simulink library "Custom_Valve_Orifices_Lib"  (R2013a)
settings: Solver=ode45  SolverMode=SingleTasking  StartTime=0.0  StopTime=10.0  RelTol=1e-3
libraries: fl_lib x20, sh_lib x13, nesl_utility x10, Custom_Valve_Orifices_Lib x1
Description:
  | Copyright 2013 The MathWorks, Inc.
settings Model: Creator=smiller  LastModifiedBy=smiller

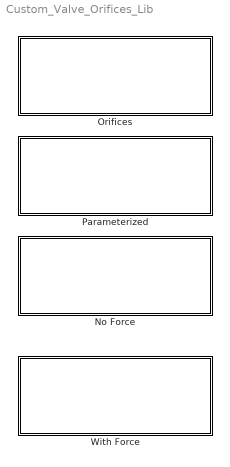
== system Custom_Valve_Orifices_Lib ==
  No Force : Subsystem  mask(Valve Orifices){or_width=24.5, x0_PA=0, x0_PB=0, x0_AT=0, x0_BT=0}
      mask prompts: or_width "Orifice Width (mm):"; x0_PA "Initial Opening PA (mm):"; x0_PB "Initial Opening PB (mm):"; x0_AT "Initial Opening AT (mm):"; x0_BT "Initial Opening BT (mm):"
      mask help: Orifice configuration for 4-way directional valve.
      mask Display: image(imread('Custom_Valve_Orifices_No_Force.jpg'));
  Orifices : Subsystem  BlockChoice=No Force
      settings: TemplateBlock=self  MemberBlocks=No Force,Parameterized,With Force
  Parameterized : Subsystem  mask(Valve Orifices){or_width=24.5, max_sp_trv=0.005, x0_PA=0, x0_PB=0, x0_AT=0, x0_BT=0}
      mask prompts: or_width "Orifice Width (mm):"; max_sp_trv "Max Orifice Length (m):"; x0_PA "Initial Opening PA (mm):"; x0_PB "Initial Opening PB (mm):"; x0_AT "Initial Opening AT (mm):"; x0_BT "Initial Opening BT (mm):"
      mask help: Orifice configuration for 4-way directional valve.
      mask Display:
      | plot([0;337.311462499201;337.311462499201;0;0], [566.910021007061;566.910021007061;0;0;566.910021007061])
      | plot([84.6585631370544;241.503668949008], [363.200353458524;363.200353458524])
      | plot([84.6585631370544;241.503668949008], [204.843487590551;204.843487590551])
      | plot([84.6585631370544;241.503668949008;241.503668949008;84.6585631370544;84.6585631370544], [521.494229324162;521.494229324162;46.486621722579;46.486621722579;521.494229324162])
      | plot([84.6585631370544;241.503668949008], [479.353917762637;479.353917762637])
      | patch([241.503668949008;197.47365731746;197.47365731746;241.503668949008], [479.353917762637;489.936238154769;468.771597370505;479.353917762637], [0;0;0])
      | plot([241.503668949008;197.47365731746;197.47365731746;241.503668949008], [479.353917762637;489.936238154769;468.771597370505;479.353917762637])
      | patch([84.6585631370544;128.562594763935;128.562594763935;84.6585631370544], [405.403655022383;415.985975414515;394.821334630251;405.403655022383], [0;0;0])
      | plot([84.6585631370544;128.562594763935;128.562594763935;84.6585631370544], [405.403655022383;415.985975414515;394.821334630251;405.403655022383])
      | plot([241.503668949008;210.071657784283], [320.997051894665;320.997051894665])
      | plot([210.071657784283;210.071657784283;210.071657784283], [336.807542480528;305.186561308801;310.414731502533])
      | plot([241.503668949008;210.071657784283], [247.04678915441;247.04678915441])
      | plot([210.071657784283;210.071657784283;210.071657784283], [262.857279740274;231.236298568547;236.464468762279])
      | plot([84.6585631370544;115.964594297111], [247.04678915441;247.04678915441])
      | plot([115.964594297111;115.964594297111;115.964594297111], [262.857279740274;231.236298568547;236.464468762279])
      | plot([84.6585631370544;115.964594297111], [320.997051894665;320.997051894665])
      | plot([115.964594297111;115.964594297111;115.964594297111], [336.807542480528;305.186561308801;310.414731502533])
      | plot([84.6585631370544;241.503668949008], [175.868086516857;80.2492629736662])
      | plot([241.503668949008;84.6585631370544], [173.474466428161;80.2492629736662])
      | plot([84.6585631370544;241.503668949008], [405.403655022383;405.403655022383])
      | patch([85.0365031510592;110.547454096377;121.885654516518;85.0365031510592], [82.2019530460238;110.547454096377;90.7056033611298;82.2019530460238], [0;0;0])
      | plot([85.0365031510592;110.547454096377;121.885654516518;85.0365031510592], [82.2019530460238;110.547454096377;90.7056033611298;82.2019530460238])
      | patch([240.936758928001;204.087607562542;215.425807982683;240.936758928001], [79.3674029409885;90.7056033611298;110.547454096377;79.3674029409885], [0;0;0])
      | plot([240.936758928001;204.087607562542;215.425807982683;240.936758928001], [79.3674029409885;90.7056033611298;110.547454096377;79.3674029409885])
  With Force : Subsystem  mask(Valve Orifices, Forces){or_width=24.5, x0_PA=0, x0_PB=0, x0_AT=0, x0_BT=0, rad_clearance=0.05}
      mask prompts: or_width "Orifice Width (mm):"; x0_PA "Initial Opening PA (mm):"; x0_PB "Initial Opening PB (mm):"; x0_AT "Initial Opening AT (mm):"; x0_BT "Initial Opening BT (mm):"; rad_clearance "Spool Radial Clearance (mm):"
      mask help: Orifice configuration for 4-way directional valve with hydraulic forces.
      mask Display: image(imread('Custom_Valve_Orifices_With_Force.jpg'));

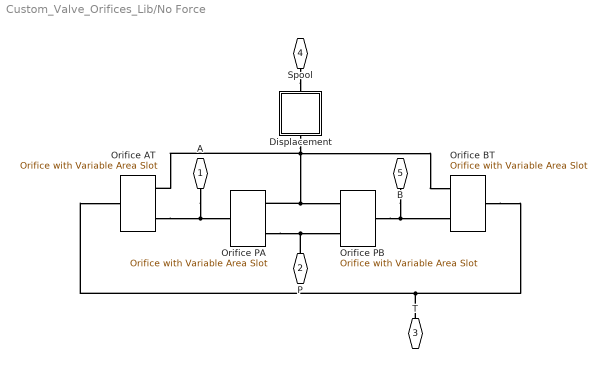
== system Custom_Valve_Orifices_Lib/No Force ==
  Displacement : Subsystem
      mask Display:
      | plot([311.800511553884;0;0;311.800511553884;311.800511553884], [311.800511553884;311.800511553884;0;0;311.800511553884])
      | plot([25.5109509453177;56.6910021007061;70.8637526258826;96.3747035712004;127.554754726589;155.900255776942;184.245756827295;212.591257877648;235.26765871793;252.274959348142;283.455010503531], [155.900255776942;155.900255776942;110.547454096377;198.418507352471;113.382004201412;198.418507352471;116.216554306448;198.418507352471;113.382004201412;155.900255776942;155.900255776942])
      | plot([155.900255776942;155.900255776942], [266.447709873319;198.418507352471])
      | patch([155.900255776942;170.073006302118;141.727505251765;155.900255776942], [198.418507352471;226.764008402824;226.764008402824;198.418507352471], [0;0;0])
      | plot([155.900255776942;170.073006302118;141.727505251765;155.900255776942], [198.418507352471;226.764008402824;226.764008402824;198.418507352471])
  Orifice AT : sh_lib/Orifices/Orifice with Variable Area Slot  Tag=Factory Generic  w=or_width mm  C_d=0.7  x_0=x0_AT mm  or=2  Re_cr=12  A_leak=1e-9 m^2  flow_rate_Log=off  pr_drop_Log=off  Re_Log=off  orif_opening_Log=off  power_Log=off  LocalVarNames=|flow_rate|pr_drop|Re|orif_opening|power  LocalVarDescs=|Flow rate through the orifice (m^3)|Pressure drop across the orifice (Pa)|Reynolds number|Orifice opening (m)|Power dissipated in the orifice (W)  LocalVarLogging=[0 0 0 0 0]
  Orifice BT : sh_lib/Orifices/Orifice with Variable Area Slot  Tag=Factory Generic  w=or_width mm  C_d=0.7  x_0=x0_BT mm  or=1  Re_cr=12  A_leak=1e-9 m^2  flow_rate_Log=off  pr_drop_Log=off  Re_Log=off  orif_opening_Log=off  power_Log=off  LocalVarNames=|flow_rate|pr_drop|Re|orif_opening|power  LocalVarDescs=|Flow rate through the orifice (m^3)|Pressure drop across the orifice (Pa)|Reynolds number|Orifice opening (m)|Power dissipated in the orifice (W)  LocalVarLogging=[0 0 0 0 0]
  Orifice PA : sh_lib/Orifices/Orifice with Variable Area Slot  Tag=Factory Generic  w=or_width mm  C_d=0.7  x_0=x0_PA mm  or=1  Re_cr=12  A_leak=1e-9 m^2  flow_rate_Log=off  pr_drop_Log=off  Re_Log=off  orif_opening_Log=off  power_Log=off  LocalVarNames=|flow_rate|pr_drop|Re|orif_opening|power  LocalVarDescs=|Flow rate through the orifice (m^3)|Pressure drop across the orifice (Pa)|Reynolds number|Orifice opening (m)|Power dissipated in the orifice (W)  LocalVarLogging=[0 0 0 0 0]
  Orifice PB : sh_lib/Orifices/Orifice with Variable Area Slot  Tag=Factory Generic  w=or_width mm  C_d=0.7  x_0=x0_PB mm  or=2  Re_cr=12  A_leak=1e-9 m^2  flow_rate_Log=off  pr_drop_Log=off  Re_Log=off  orif_opening_Log=off  power_Log=off  LocalVarNames=|flow_rate|pr_drop|Re|orif_opening|power  LocalVarDescs=|Flow rate through the orifice (m^3)|Pressure drop across the orifice (Pa)|Reynolds number|Orifice opening (m)|Power dissipated in the orifice (W)  LocalVarLogging=[0 0 0 0 0]
  A : PMIOPort  Port=1  Side=Right
  P : PMIOPort  Port=2  Side=Left
  T : PMIOPort  Port=3  Side=Left
  Spool : PMIOPort  Port=4  Side=Right
  B : PMIOPort  Port=5  Side=Right
  connections:
  Orifice PB/RConn1 -- B/RConn1 -- Orifice BT/LConn2
  Orifice BT/RConn1 -- Orifice AT/RConn1 -- T/RConn1
  A/RConn1 -- Orifice PA/RConn1 -- Orifice AT/LConn2
  P/RConn1 -- Orifice PB/LConn2 -- Orifice PA/LConn2
  Displacement/RConn1 -- Orifice BT/LConn1 -- Orifice PB/LConn1 -- Orifice PA/LConn1 -- Orifice AT/LConn1
  Spool/RConn1 -- Displacement/LConn1

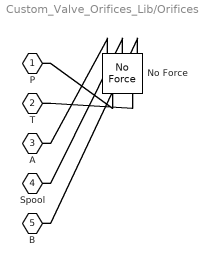
== system Custom_Valve_Orifices_Lib/Orifices ==
  No Force : Custom_Valve_Orifices_Lib/No Force  or_width=24.5  x0_PA=0  x0_PB=0  x0_AT=0  x0_BT=0
  P : PMIOPort  Port=1  Side=Left
  T : PMIOPort  Port=2  Side=Left
  A : PMIOPort  Port=3  Side=Right
  Spool : PMIOPort  Port=4  Side=Right
  B : PMIOPort  Port=5  Side=Right
  connections:
  No Force/LConn1 -- P/RConn1
  No Force/LConn2 -- T/RConn1
  No Force/RConn1 -- A/RConn1
  No Force/RConn2 -- Spool/RConn1
  No Force/RConn3 -- B/RConn1

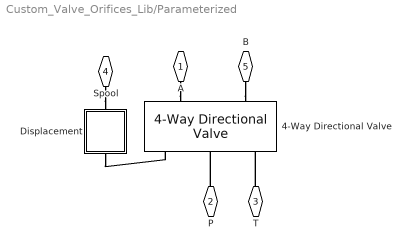
== system Custom_Valve_Orifices_Lib/Parameterized ==
  4-Way Directional Valve : sh_lib/Valves/Directional Valves/4-Way Directional Valve  mdl_type=1  area_max=or_width*max_sp_trv*1e3 mm^2  opening_max=max_sp_trv m  opening_tab="[  -0.002 0 0.002 0.005 0.015 ] m"  area_tab="[  1e-09 2.0352e-07 4.0736e-05 0.00011438 0.00034356 ] m^2"  pressure_tab="[  -1e+07 -5e+06 -2e+06 2e+06 5e+06 1e+07 ] Pa"  flow_rate_tab="[  -1e-07 -7.0711e-08 -4.4721e-08 4.4721e-08 7.0711e-08 1e-07 ; -2.0352e-05 -1.4391e-05 -9.1017e-06 9.1017e-06 1.4391e-05 2.0352e-05 ; -0.0040736 -0.0028805 -0.0018218 0.0018218 0.0028805 0.0040736 ; -0.011438 -0.0080879 -0.0051152 0.0051152 0.0080879 0.011438 ; -0.034356 -0.024293 -0.015364 0.015364 0.024293 0.034356 ; ] m^3/s"  interp_method=1  extrap_method=1  C_d=0.7  x_0_P_A=x0_PA mm  x_0_P_B=x0_PB mm  x_0_A_T=x0_AT mm  x_0_B_T=x0_BT mm  Re_cr=12  A_leak=1e-9 m^2  LocalVarLogging=[]
  Displacement : Subsystem
      mask Display:
      | plot([311.800511553884;0;0;311.800511553884;311.800511553884], [311.800511553884;311.800511553884;0;0;311.800511553884])
      | plot([25.5109509453177;56.6910021007061;70.8637526258826;96.3747035712004;127.554754726589;155.900255776942;184.245756827295;212.591257877648;235.26765871793;252.274959348142;283.455010503531], [155.900255776942;155.900255776942;110.547454096377;198.418507352471;113.382004201412;198.418507352471;116.216554306448;198.418507352471;113.382004201412;155.900255776942;155.900255776942])
      | plot([155.900255776942;155.900255776942], [266.447709873319;198.418507352471])
      | patch([155.900255776942;170.073006302118;141.727505251765;155.900255776942], [198.418507352471;226.764008402824;226.764008402824;198.418507352471], [0;0;0])
      | plot([155.900255776942;170.073006302118;141.727505251765;155.900255776942], [198.418507352471;226.764008402824;226.764008402824;198.418507352471])
  A : PMIOPort  Port=1  Side=Right
  P : PMIOPort  Port=2  Side=Left
  T : PMIOPort  Port=3  Side=Left
  Spool : PMIOPort  Port=4  Side=Right
  B : PMIOPort  Port=5  Side=Right
  connections:
  Displacement/RConn1 -- 4-Way Directional Valve/RConn1
  P/RConn1 -- 4-Way Directional Valve/RConn2
  A/RConn1 -- 4-Way Directional Valve/LConn1
  B/RConn1 -- 4-Way Directional Valve/LConn2
  T/RConn1 -- 4-Way Directional Valve/RConn3
  Spool/RConn1 -- Displacement/LConn1

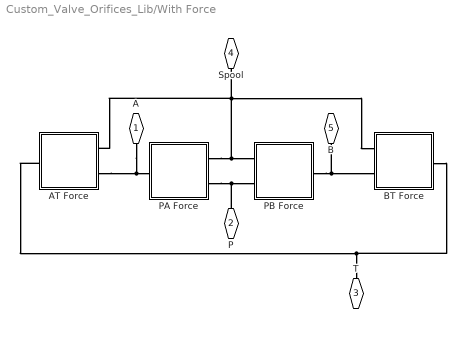
== system Custom_Valve_Orifices_Lib/With Force ==
  AT Force : Subsystem
  BT Force : Subsystem
  PA Force : Subsystem
  PB Force : Subsystem
  A : PMIOPort  Port=1  Side=Right
  P : PMIOPort  Port=2  Side=Left
  T : PMIOPort  Port=3  Side=Left
  Spool : PMIOPort  Port=4  Side=Right
  B : PMIOPort  Port=5  Side=Right
  connections:
  PA Force/LConn1 -- PB Force/LConn1 -- BT Force/LConn1 -- Spool/RConn1 -- AT Force/LConn1
  PA Force/LConn2 -- PB Force/LConn2 -- P/RConn1
  PA Force/RConn1 -- AT Force/LConn2 -- A/RConn1
  AT Force/RConn1 -- BT Force/RConn1 -- T/RConn1
  PB Force/RConn1 -- BT Force/LConn2 -- B/RConn1

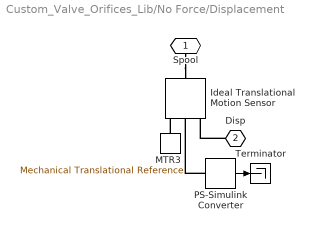
== system Custom_Valve_Orifices_Lib/No Force/Displacement ==
  Ideal Translational Motion Sensor : fl_lib/Mechanical/Mechanical Sensors/Ideal Translational Motion Sensor  Tag=Factory Generic  offset=0 m  v_Log=off  f_Log=off  x_Log=off  LocalVarNames=|v|f|x  LocalVarDescs=|v|f|x  LocalVarLogging=[]
  MTR3 : fl_lib/Mechanical/Translational Elements/Mechanical Translational Reference  Tag=Factory Generic  SystemSampleTime=-1  LocalVarLogging=[]
  PS-Simulink Converter : nesl_utility/PS-Simulink Converter  SystemSampleTime=-1  PhysicalDomain=network_engine_domain  LeftPortType=input  RightPortType=output  SubClassName=ps_output  Unit=1  AffineConversion=off
  Terminator : Terminator
  Spool : PMIOPort  Port=1  Side=Left
  Disp : PMIOPort  Port=2  Side=Right
  wires:
  PS-Simulink Converter/1 -> Terminator/1
  connections:
  MTR3/LConn1 -- Ideal Translational Motion Sensor/RConn1
  PS-Simulink Converter/LConn1 -- Ideal Translational Motion Sensor/RConn2
  Spool/RConn1 -- Ideal Translational Motion Sensor/LConn1
  Disp/RConn1 -- Ideal Translational Motion Sensor/RConn3

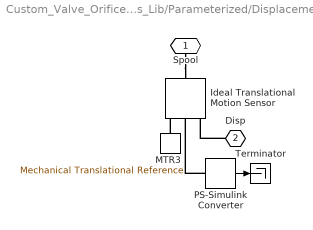
== system Custom_Valve_Orifices_Lib/Parameterized/Displacement ==
  Ideal Translational Motion Sensor : fl_lib/Mechanical/Mechanical Sensors/Ideal Translational Motion Sensor  Tag=Factory Generic  offset=0 m  v_Log=off  f_Log=off  x_Log=off  LocalVarNames=|v|f|x  LocalVarDescs=|v|f|x  LocalVarLogging=[]
  MTR3 : fl_lib/Mechanical/Translational Elements/Mechanical Translational Reference  Tag=Factory Generic  SystemSampleTime=-1  LocalVarLogging=[]
  PS-Simulink Converter : nesl_utility/PS-Simulink Converter  SystemSampleTime=-1  PhysicalDomain=network_engine_domain  LeftPortType=input  RightPortType=output  SubClassName=ps_output  Unit=1  AffineConversion=off
  Terminator : Terminator
  Spool : PMIOPort  Port=1  Side=Left
  Disp : PMIOPort  Port=2  Side=Right
  wires:
  PS-Simulink Converter/1 -> Terminator/1
  connections:
  Disp/RConn1 -- Ideal Translational Motion Sensor/RConn3
  Spool/RConn1 -- Ideal Translational Motion Sensor/LConn1
  PS-Simulink Converter/LConn1 -- Ideal Translational Motion Sensor/RConn2
  MTR3/LConn1 -- Ideal Translational Motion Sensor/RConn1

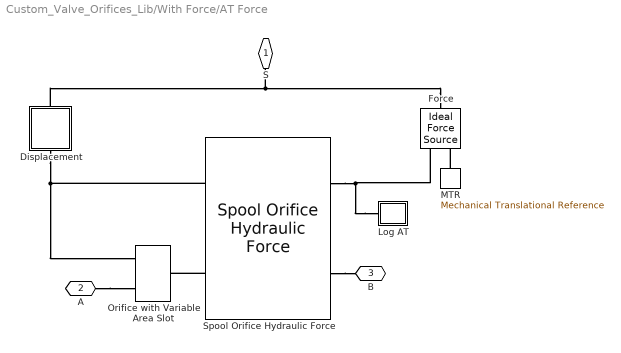
== system Custom_Valve_Orifices_Lib/With Force/AT Force ==
  Displacement : Subsystem
      mask Display:
      | plot([311.800511553884;0;0;311.800511553884;311.800511553884], [311.800511553884;311.800511553884;0;0;311.800511553884])
      | plot([25.5109509453177;56.6910021007061;70.8637526258826;96.3747035712004;127.554754726589;155.900255776942;184.245756827295;212.591257877648;235.26765871793;252.274959348142;283.455010503531], [155.900255776942;155.900255776942;110.547454096377;198.418507352471;113.382004201412;198.418507352471;116.216554306448;198.418507352471;113.382004201412;155.900255776942;155.900255776942])
      | plot([155.900255776942;155.900255776942], [266.447709873319;198.418507352471])
      | patch([155.900255776942;170.073006302118;141.727505251765;155.900255776942], [198.418507352471;226.764008402824;226.764008402824;198.418507352471], [0;0;0])
      | plot([155.900255776942;170.073006302118;141.727505251765;155.900255776942], [198.418507352471;226.764008402824;226.764008402824;198.418507352471])
  Force : fl_lib/Mechanical/Mechanical Sources/Ideal Force Source  Tag=Factory Generic  v_Log=off  f_Log=off  LocalVarNames=|force|rel_velocity|power  LocalVarDescs=|Force (N)|Relative velocity (m/s)|Power generated by the source (W)  LocalVarLogging=[0 0 0]
  Log AT : Subsystem
  MTR : fl_lib/Mechanical/Translational Elements/Mechanical Translational Reference  Tag=Factory Generic  f_Log=off  LocalVarNames=|f  LocalVarDescs=|f  LocalVarLogging=[]
  Orifice with Variable Area Slot : sh_lib/Orifices/Orifice with Variable Area Slot  Tag=Factory Generic  w=or_width mm  C_d=0.7  x_0=x0_AT mm  or=2  Re_cr=12  A_leak=1e-9 m^2  flow_rate_Log=off  pr_drop_Log=off  Re_Log=off  orif_opening_Log=off  power_Log=off  LocalVarNames=|flow_rate|pr_drop|Re|orif_opening|power  LocalVarDescs=|Flow rate through the orifice (m^3)|Pressure drop across the orifice (Pa)|Reynolds number|Orifice opening (m)|Power dissipated in the orifice (W)  LocalVarLogging=[0 0 0 0 0]
  Spool Orifice Hydraulic Force : sh_lib/Valves/Valve Forces/Spool Orifice Hydraulic Force  or_type=1  w=or_width mm  rad_clear=rad_clearance mm  or_diam=0.005 m  or_numb=4  x_0=x0_AT mm  or=2  flow_rate_Log=off  opening_Log=off  area_Log=off  jet_angle_Log=off  axial_force_Log=off  LocalVarNames=|flow_rate|opening|area|jet_angle|axial_force  LocalVarDescs=|Flow rate through the orifice (m^3/s)|Orifice opening (m)|Orifice area (m^3)|Jet angle (deg)|Hydraulic axial force (N)  LocalVarLogging=[0 0 0 0 0]
  S : PMIOPort  Port=1  Side=Left
  A : PMIOPort  Port=2  Side=Left
  B : PMIOPort  Port=3  Side=Right
  connections:
  Displacement/RConn1 -- Spool Orifice Hydraulic Force/LConn2 -- Orifice with Variable Area Slot/LConn1
  Force/LConn1 -- S/RConn1 -- Displacement/LConn1
  MTR/LConn1 -- Force/RConn2
  Spool Orifice Hydraulic Force/RConn1 -- B/RConn1
  Spool Orifice Hydraulic Force/LConn1 -- Orifice with Variable Area Slot/RConn1
  A/RConn1 -- Orifice with Variable Area Slot/LConn2
  Log AT/LConn1 -- Spool Orifice Hydraulic Force/RConn2 -- Force/RConn1

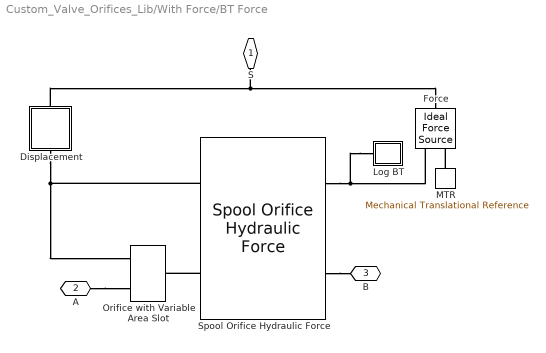
== system Custom_Valve_Orifices_Lib/With Force/BT Force ==
  Displacement : Subsystem
      mask Display:
      | plot([311.800511553884;0;0;311.800511553884;311.800511553884], [311.800511553884;311.800511553884;0;0;311.800511553884])
      | plot([25.5109509453177;56.6910021007061;70.8637526258826;96.3747035712004;127.554754726589;155.900255776942;184.245756827295;212.591257877648;235.26765871793;252.274959348142;283.455010503531], [155.900255776942;155.900255776942;110.547454096377;198.418507352471;113.382004201412;198.418507352471;116.216554306448;198.418507352471;113.382004201412;155.900255776942;155.900255776942])
      | plot([155.900255776942;155.900255776942], [266.447709873319;198.418507352471])
      | patch([155.900255776942;170.073006302118;141.727505251765;155.900255776942], [198.418507352471;226.764008402824;226.764008402824;198.418507352471], [0;0;0])
      | plot([155.900255776942;170.073006302118;141.727505251765;155.900255776942], [198.418507352471;226.764008402824;226.764008402824;198.418507352471])
  Force : fl_lib/Mechanical/Mechanical Sources/Ideal Force Source  Tag=Factory Generic  v_Log=off  f_Log=off  LocalVarNames=|force|rel_velocity|power  LocalVarDescs=|Force (N)|Relative velocity (m/s)|Power generated by the source (W)  LocalVarLogging=[0 0 0]
  Log BT : Subsystem
  MTR : fl_lib/Mechanical/Translational Elements/Mechanical Translational Reference  Tag=Factory Generic  f_Log=off  LocalVarNames=|f  LocalVarDescs=|f  LocalVarLogging=[]
  Orifice with Variable Area Slot : sh_lib/Orifices/Orifice with Variable Area Slot  Tag=Factory Generic  w=or_width mm  C_d=0.7  x_0=x0_BT mm  or=1  Re_cr=12  A_leak=1e-9 m^2  flow_rate_Log=off  pr_drop_Log=off  Re_Log=off  orif_opening_Log=off  power_Log=off  LocalVarNames=|flow_rate|pr_drop|Re|orif_opening|power  LocalVarDescs=|Flow rate through the orifice (m^3)|Pressure drop across the orifice (Pa)|Reynolds number|Orifice opening (m)|Power dissipated in the orifice (W)  LocalVarLogging=[0 0 0 0 0]
  Spool Orifice Hydraulic Force : sh_lib/Valves/Valve Forces/Spool Orifice Hydraulic Force  or_type=1  w=or_width mm  rad_clear=rad_clearance mm  or_diam=0.005 m  or_numb=4  x_0=x0_BT mm  or=1  flow_rate_Log=off  opening_Log=off  area_Log=off  jet_angle_Log=off  axial_force_Log=off  LocalVarNames=|flow_rate|opening|area|jet_angle|axial_force  LocalVarDescs=|Flow rate through the orifice (m^3/s)|Orifice opening (m)|Orifice area (m^3)|Jet angle (deg)|Hydraulic axial force (N)  LocalVarLogging=[0 0 0 0 0]
  S : PMIOPort  Port=1  Side=Left
  A : PMIOPort  Port=2  Side=Left
  B : PMIOPort  Port=3  Side=Right
  connections:
  Displacement/RConn1 -- Spool Orifice Hydraulic Force/LConn2 -- Orifice with Variable Area Slot/LConn1
  S/RConn1 -- Force/LConn1 -- Displacement/LConn1
  MTR/LConn1 -- Force/RConn2
  Spool Orifice Hydraulic Force/RConn1 -- B/RConn1
  Spool Orifice Hydraulic Force/LConn1 -- Orifice with Variable Area Slot/RConn1
  A/RConn1 -- Orifice with Variable Area Slot/LConn2
  Log BT/LConn1 -- Spool Orifice Hydraulic Force/RConn2 -- Force/RConn1

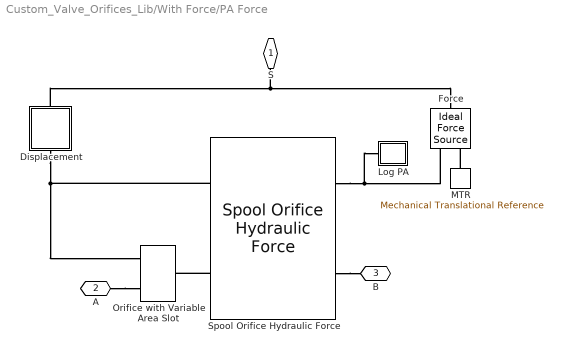
== system Custom_Valve_Orifices_Lib/With Force/PA Force ==
  Displacement : Subsystem
      mask Display:
      | plot([311.800511553884;0;0;311.800511553884;311.800511553884], [311.800511553884;311.800511553884;0;0;311.800511553884])
      | plot([25.5109509453177;56.6910021007061;70.8637526258826;96.3747035712004;127.554754726589;155.900255776942;184.245756827295;212.591257877648;235.26765871793;252.274959348142;283.455010503531], [155.900255776942;155.900255776942;110.547454096377;198.418507352471;113.382004201412;198.418507352471;116.216554306448;198.418507352471;113.382004201412;155.900255776942;155.900255776942])
      | plot([155.900255776942;155.900255776942], [266.447709873319;198.418507352471])
      | patch([155.900255776942;170.073006302118;141.727505251765;155.900255776942], [198.418507352471;226.764008402824;226.764008402824;198.418507352471], [0;0;0])
      | plot([155.900255776942;170.073006302118;141.727505251765;155.900255776942], [198.418507352471;226.764008402824;226.764008402824;198.418507352471])
  Force : fl_lib/Mechanical/Mechanical Sources/Ideal Force Source  Tag=Factory Generic  v_Log=off  f_Log=off  LocalVarNames=|force|rel_velocity|power  LocalVarDescs=|Force (N)|Relative velocity (m/s)|Power generated by the source (W)  LocalVarLogging=[0 0 0]
  Log PA : Subsystem
  MTR : fl_lib/Mechanical/Translational Elements/Mechanical Translational Reference  Tag=Factory Generic  f_Log=off  LocalVarNames=|f  LocalVarDescs=|f  LocalVarLogging=[]
  Orifice with Variable Area Slot : sh_lib/Orifices/Orifice with Variable Area Slot  Tag=Factory Generic  w=or_width mm  C_d=0.7  x_0=x0_PA mm  or=1  Re_cr=12  A_leak=1e-9 m^2  flow_rate_Log=off  pr_drop_Log=off  Re_Log=off  orif_opening_Log=off  power_Log=off  LocalVarNames=|flow_rate|pr_drop|Re|orif_opening|power  LocalVarDescs=|Flow rate through the orifice (m^3)|Pressure drop across the orifice (Pa)|Reynolds number|Orifice opening (m)|Power dissipated in the orifice (W)  LocalVarLogging=[0 0 0 0 0]
  Spool Orifice Hydraulic Force : sh_lib/Valves/Valve Forces/Spool Orifice Hydraulic Force  or_type=1  w=or_width mm  rad_clear=rad_clearance mm  or_diam=0.005 m  or_numb=4  x_0=x0_PA mm  or=1  flow_rate_Log=off  opening_Log=off  area_Log=off  jet_angle_Log=off  axial_force_Log=off  LocalVarNames=|flow_rate|opening|area|jet_angle|axial_force  LocalVarDescs=|Flow rate through the orifice (m^3/s)|Orifice opening (m)|Orifice area (m^3)|Jet angle (deg)|Hydraulic axial force (N)  LocalVarLogging=[0 0 0 0 0]
  S : PMIOPort  Port=1  Side=Left
  A : PMIOPort  Port=2  Side=Left
  B : PMIOPort  Port=3  Side=Right
  connections:
  Log PA/LConn1 -- Spool Orifice Hydraulic Force/RConn2 -- Force/RConn1
  A/RConn1 -- Orifice with Variable Area Slot/LConn2
  Spool Orifice Hydraulic Force/LConn1 -- Orifice with Variable Area Slot/RConn1
  Spool Orifice Hydraulic Force/RConn1 -- B/RConn1
  MTR/LConn1 -- Force/RConn2
  Displacement/LConn1 -- S/RConn1 -- Force/LConn1
  Displacement/RConn1 -- Spool Orifice Hydraulic Force/LConn2 -- Orifice with Variable Area Slot/LConn1

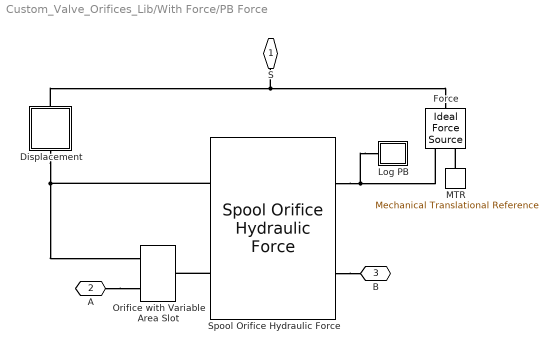
== system Custom_Valve_Orifices_Lib/With Force/PB Force ==
  Displacement : Subsystem
      mask Display:
      | plot([311.800511553884;0;0;311.800511553884;311.800511553884], [311.800511553884;311.800511553884;0;0;311.800511553884])
      | plot([25.5109509453177;56.6910021007061;70.8637526258826;96.3747035712004;127.554754726589;155.900255776942;184.245756827295;212.591257877648;235.26765871793;252.274959348142;283.455010503531], [155.900255776942;155.900255776942;110.547454096377;198.418507352471;113.382004201412;198.418507352471;116.216554306448;198.418507352471;113.382004201412;155.900255776942;155.900255776942])
      | plot([155.900255776942;155.900255776942], [266.447709873319;198.418507352471])
      | patch([155.900255776942;170.073006302118;141.727505251765;155.900255776942], [198.418507352471;226.764008402824;226.764008402824;198.418507352471], [0;0;0])
      | plot([155.900255776942;170.073006302118;141.727505251765;155.900255776942], [198.418507352471;226.764008402824;226.764008402824;198.418507352471])
  Force : fl_lib/Mechanical/Mechanical Sources/Ideal Force Source  Tag=Factory Generic  v_Log=off  f_Log=off  LocalVarNames=|force|rel_velocity|power  LocalVarDescs=|Force (N)|Relative velocity (m/s)|Power generated by the source (W)  LocalVarLogging=[0 0 0]
  Log PB : Subsystem
  MTR : fl_lib/Mechanical/Translational Elements/Mechanical Translational Reference  Tag=Factory Generic  f_Log=off  LocalVarNames=|f  LocalVarDescs=|f  LocalVarLogging=[]
  Orifice with Variable Area Slot : sh_lib/Orifices/Orifice with Variable Area Slot  Tag=Factory Generic  w=or_width mm  C_d=0.7  x_0=x0_PB mm  or=2  Re_cr=12  A_leak=1e-9 m^2  flow_rate_Log=off  pr_drop_Log=off  Re_Log=off  orif_opening_Log=off  power_Log=off  LocalVarNames=|flow_rate|pr_drop|Re|orif_opening|power  LocalVarDescs=|Flow rate through the orifice (m^3)|Pressure drop across the orifice (Pa)|Reynolds number|Orifice opening (m)|Power dissipated in the orifice (W)  LocalVarLogging=[0 0 0 0 0]
  Spool Orifice Hydraulic Force : sh_lib/Valves/Valve Forces/Spool Orifice Hydraulic Force  or_type=1  w=or_width mm  rad_clear=rad_clearance mm  or_diam=0.005 m  or_numb=4  x_0=x0_PB mm  or=2  flow_rate_Log=off  opening_Log=off  area_Log=off  jet_angle_Log=off  axial_force_Log=off  LocalVarNames=|flow_rate|opening|area|jet_angle|axial_force  LocalVarDescs=|Flow rate through the orifice (m^3/s)|Orifice opening (m)|Orifice area (m^3)|Jet angle (deg)|Hydraulic axial force (N)  LocalVarLogging=[0 0 0 0 0]
  S : PMIOPort  Port=1  Side=Left
  A : PMIOPort  Port=2  Side=Left
  B : PMIOPort  Port=3  Side=Right
  connections:
  Log PB/LConn1 -- Spool Orifice Hydraulic Force/RConn2 -- Force/RConn1
  A/RConn1 -- Orifice with Variable Area Slot/LConn2
  Spool Orifice Hydraulic Force/LConn1 -- Orifice with Variable Area Slot/RConn1
  Spool Orifice Hydraulic Force/RConn1 -- B/RConn1
  MTR/LConn1 -- Force/RConn2
  Displacement/LConn1 -- S/RConn1 -- Force/LConn1
  Displacement/RConn1 -- Spool Orifice Hydraulic Force/LConn2 -- Orifice with Variable Area Slot/LConn1

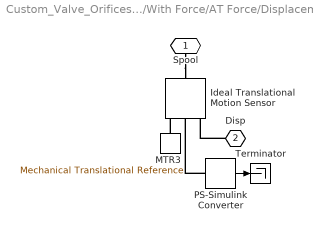
== system Custom_Valve_Orifices_Lib/With Force/AT Force/Displacement ==
  Ideal Translational Motion Sensor : fl_lib/Mechanical/Mechanical Sensors/Ideal Translational Motion Sensor  Tag=Factory Generic  offset=0 m  v_Log=off  f_Log=off  x_Log=off  LocalVarNames=|v|f|x  LocalVarDescs=|v|f|x  LocalVarLogging=[]
  MTR3 : fl_lib/Mechanical/Translational Elements/Mechanical Translational Reference  Tag=Factory Generic  SystemSampleTime=-1  LocalVarLogging=[]
  PS-Simulink Converter : nesl_utility/PS-Simulink Converter  SystemSampleTime=-1  PhysicalDomain=network_engine_domain  LeftPortType=input  RightPortType=output  SubClassName=ps_output  Unit=1  AffineConversion=off
  Terminator : Terminator
  Spool : PMIOPort  Port=1  Side=Left
  Disp : PMIOPort  Port=2  Side=Right
  wires:
  PS-Simulink Converter/1 -> Terminator/1
  connections:
  Disp/RConn1 -- Ideal Translational Motion Sensor/RConn3
  Spool/RConn1 -- Ideal Translational Motion Sensor/LConn1
  PS-Simulink Converter/LConn1 -- Ideal Translational Motion Sensor/RConn2
  MTR3/LConn1 -- Ideal Translational Motion Sensor/RConn1

== system Custom_Valve_Orifices_Lib/With Force/AT Force/Log AT ==
  PS-Simulink Converter : nesl_utility/PS-Simulink Converter  PhysicalDomain=network_engine_domain  SubClassName=ps_output  LeftPortType=input  RightPortType=output  PseudoPeriodic=off  Frequencies=[]  Unit=1  AffineConversion=off
  To Workspace : ToWorkspace  VariableName=Spool_Hydr_Force_AT  SampleTime=-1  SaveFormat=Structure With Time
  Log : PMIOPort  Port=1  Side=Left
  wires:
  PS-Simulink Converter/1 -> To Workspace/1
  connections:
  Log/RConn1 -- PS-Simulink Converter/LConn1

== system Custom_Valve_Orifices_Lib/With Force/BT Force/Displacement ==
  Ideal Translational Motion Sensor : fl_lib/Mechanical/Mechanical Sensors/Ideal Translational Motion Sensor  Tag=Factory Generic  offset=0 m  v_Log=off  f_Log=off  x_Log=off  LocalVarNames=|v|f|x  LocalVarDescs=|v|f|x  LocalVarLogging=[]
  MTR3 : fl_lib/Mechanical/Translational Elements/Mechanical Translational Reference  Tag=Factory Generic  SystemSampleTime=-1  LocalVarLogging=[]
  PS-Simulink Converter : nesl_utility/PS-Simulink Converter  SystemSampleTime=-1  PhysicalDomain=network_engine_domain  LeftPortType=input  RightPortType=output  SubClassName=ps_output  Unit=1  AffineConversion=off
  Terminator : Terminator
  Spool : PMIOPort  Port=1  Side=Left
  Disp : PMIOPort  Port=2  Side=Right
  wires:
  PS-Simulink Converter/1 -> Terminator/1
  connections:
  Disp/RConn1 -- Ideal Translational Motion Sensor/RConn3
  Spool/RConn1 -- Ideal Translational Motion Sensor/LConn1
  PS-Simulink Converter/LConn1 -- Ideal Translational Motion Sensor/RConn2
  MTR3/LConn1 -- Ideal Translational Motion Sensor/RConn1

== system Custom_Valve_Orifices_Lib/With Force/BT Force/Log BT ==
  PS-Simulink Converter : nesl_utility/PS-Simulink Converter  PhysicalDomain=network_engine_domain  SubClassName=ps_output  LeftPortType=input  RightPortType=output  PseudoPeriodic=off  Frequencies=[]  Unit=1  AffineConversion=off
  To Workspace : ToWorkspace  VariableName=Spool_Hydr_Force_BT  SampleTime=-1  SaveFormat=Structure With Time
  Log : PMIOPort  Port=1  Side=Left
  wires:
  PS-Simulink Converter/1 -> To Workspace/1
  connections:
  Log/RConn1 -- PS-Simulink Converter/LConn1

== system Custom_Valve_Orifices_Lib/With Force/PA Force/Displacement ==
  Ideal Translational Motion Sensor : fl_lib/Mechanical/Mechanical Sensors/Ideal Translational Motion Sensor  Tag=Factory Generic  offset=0 m  v_Log=off  f_Log=off  x_Log=off  LocalVarNames=|v|f|x  LocalVarDescs=|v|f|x  LocalVarLogging=[]
  MTR3 : fl_lib/Mechanical/Translational Elements/Mechanical Translational Reference  Tag=Factory Generic  SystemSampleTime=-1  LocalVarLogging=[]
  PS-Simulink Converter : nesl_utility/PS-Simulink Converter  SystemSampleTime=-1  PhysicalDomain=network_engine_domain  LeftPortType=input  RightPortType=output  SubClassName=ps_output  Unit=1  AffineConversion=off
  Terminator : Terminator
  Spool : PMIOPort  Port=1  Side=Left
  Disp : PMIOPort  Port=2  Side=Right
  wires:
  PS-Simulink Converter/1 -> Terminator/1
  connections:
  MTR3/LConn1 -- Ideal Translational Motion Sensor/RConn1
  PS-Simulink Converter/LConn1 -- Ideal Translational Motion Sensor/RConn2
  Spool/RConn1 -- Ideal Translational Motion Sensor/LConn1
  Disp/RConn1 -- Ideal Translational Motion Sensor/RConn3

== system Custom_Valve_Orifices_Lib/With Force/PA Force/Log PA ==
  PS-Simulink Converter : nesl_utility/PS-Simulink Converter  PhysicalDomain=network_engine_domain  SubClassName=ps_output  LeftPortType=input  RightPortType=output  PseudoPeriodic=off  Frequencies=[]  Unit=1  AffineConversion=off
  To Workspace : ToWorkspace  VariableName=Spool_Hydr_Force_PA  SampleTime=-1  SaveFormat=Structure With Time
  Log : PMIOPort  Port=1  Side=Left
  wires:
  PS-Simulink Converter/1 -> To Workspace/1
  connections:
  Log/RConn1 -- PS-Simulink Converter/LConn1

== system Custom_Valve_Orifices_Lib/With Force/PB Force/Displacement ==
  Ideal Translational Motion Sensor : fl_lib/Mechanical/Mechanical Sensors/Ideal Translational Motion Sensor  Tag=Factory Generic  offset=0 m  v_Log=off  f_Log=off  x_Log=off  LocalVarNames=|v|f|x  LocalVarDescs=|v|f|x  LocalVarLogging=[]
  MTR3 : fl_lib/Mechanical/Translational Elements/Mechanical Translational Reference  Tag=Factory Generic  SystemSampleTime=-1  LocalVarLogging=[]
  PS-Simulink Converter : nesl_utility/PS-Simulink Converter  SystemSampleTime=-1  PhysicalDomain=network_engine_domain  LeftPortType=input  RightPortType=output  SubClassName=ps_output  Unit=1  AffineConversion=off
  Terminator : Terminator
  Spool : PMIOPort  Port=1  Side=Left
  Disp : PMIOPort  Port=2  Side=Right
  wires:
  PS-Simulink Converter/1 -> Terminator/1
  connections:
  MTR3/LConn1 -- Ideal Translational Motion Sensor/RConn1
  PS-Simulink Converter/LConn1 -- Ideal Translational Motion Sensor/RConn2
  Spool/RConn1 -- Ideal Translational Motion Sensor/LConn1
  Disp/RConn1 -- Ideal Translational Motion Sensor/RConn3

== system Custom_Valve_Orifices_Lib/With Force/PB Force/Log PB ==
  PS-Simulink Converter : nesl_utility/PS-Simulink Converter  PhysicalDomain=network_engine_domain  SubClassName=ps_output  LeftPortType=input  RightPortType=output  PseudoPeriodic=off  Frequencies=[]  Unit=1  AffineConversion=off
  To Workspace : ToWorkspace  VariableName=Spool_Hydr_Force_PB  SampleTime=-1  SaveFormat=Structure With Time
  Log : PMIOPort  Port=1  Side=Left
  wires:
  PS-Simulink Converter/1 -> To Workspace/1
  connections:
  Log/RConn1 -- PS-Simulink Converter/LConn1
